simulink model "feedback_plant"  (R2024a)
settings: Solver=FixedStepAuto  StartTime=0.0  StopTime=Inf  FixedStep=5e-6  MaxStep=0.1  RelTol=1e-3  EnableMultiTasking=on
libraries: simulink x2
settings Model: ModifiedByFormat=The MathWorks Inc.  ExtModeTrigDuration=8  Creator=The MathWorks, Inc.  LastModifiedBy=The MathWorks Inc.
settings SolverCC: AlgebraicLoopSolver=TrustRegion
settings DataIOCC: SaveFormat=Array  ReturnWorkspaceOutputs=off
settings OptimizationCC: DefaultUnderspecifiedDataType=single  EnhancedBackFolding=on  PassReuseOutputArgsAs=Individual arguments  ExpressionDepthLimit=2147483647  MaxStackSize=1024  OptimizeBlockOrder=speed  DifferentSizesBufferReuse=on  OptimizationCustomize=off  EfficientTunableParamExpr=on
settings DebuggingCC: UnderspecifiedInitializationDetection=Classic  MergeDetectMultiDrivingBlocksExec=none  SolverPrmCheckMsg=warning  ParameterTunabilityLossMsg=error  FcnCallInpInsideContextMsg=warning  UnconnectedInputMsg=warning  UnconnectedOutputMsg=warning  UnconnectedLineMsg=warning  AllowSymbolicDim=off  StateNameClashWarn=warning  SFUnexpectedBacktrackingDiag=warning  SFNoUnconditionalDefaultTransitionDiag=warning  SFExecutionAtInitializationDiag=none  ArithmeticOperatorsInVariantConditions=warning
settings HardwareCC: ProdBitPerChar=16  ProdBitPerInt=16  ProdBitPerPointer=32  ProdBitPerSizeT=32  ProdBitPerPtrDiffT=32  ProdLargestAtomicInteger=Integer  ProdLargestAtomicFloat=None  ProdWordSize=16  ProdLongLongMode=on  ProdHWDeviceType=Texas Instruments->C2000  HardwareBoardFeatureSet=SoCBlockset
settings ModelReferenceCC: EnableRefExpFcnMdlSchedulingChecks=on  PropagateSignalLabelsOutOfModel=off
settings SFSimCC: SimUseLocalCustomCode=off  MATLABDynamicMemAlloc=off  CustomCodeUndefinedFunction=UseInterfaceOnly
settings RTWCC: Description=Embedded Coder  SystemTargetFile=ert.tlc  HardwareBoard=TI Delfino F28379D LaunchPad  TemplateMakefile=ert_default_tmf  RTWUseLocalCustomCode=off  Toolchain=Texas Instruments Code Composer Studio (C2000)  CodeProfilingSaveOptions=MetricsOnly  GPUComputeCapability=3.5
settings CodeAppCC: ForceParamTrailComments=on  IgnoreCustomStorageClasses=off  OperatorAnnotations=on  SimulinkDataObjDesc=on  SFDataObjDesc=on  InsertBlockDesc=on
settings ERTTargetCC: CodeReplacementLibrary=TI C28x  SupportContinuousTime=on  ExtModeTransport=4  ExtModeStaticAlloc=on  ExtModeAutomaticAllocSize=off  ExtModeStaticAllocSize=10000  ExtModeMexFile=ext_xcp  ExtModeIntrfLevel=Level2 - Open
settings ConfigComp: CovMetricSettings=dw  CovSaveCumulativeToWorkspaceVar=on  CovSaveSingleToWorkspaceVar=on  CovExternalEMLEnable=off  CovSFcnEnable=off

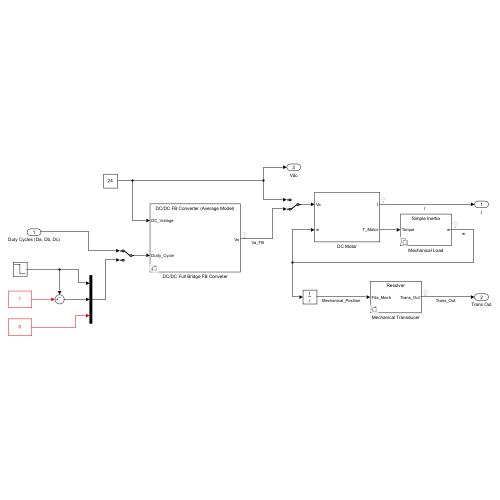
[thumbnail: Simulink's stored preview of the top-level diagram]
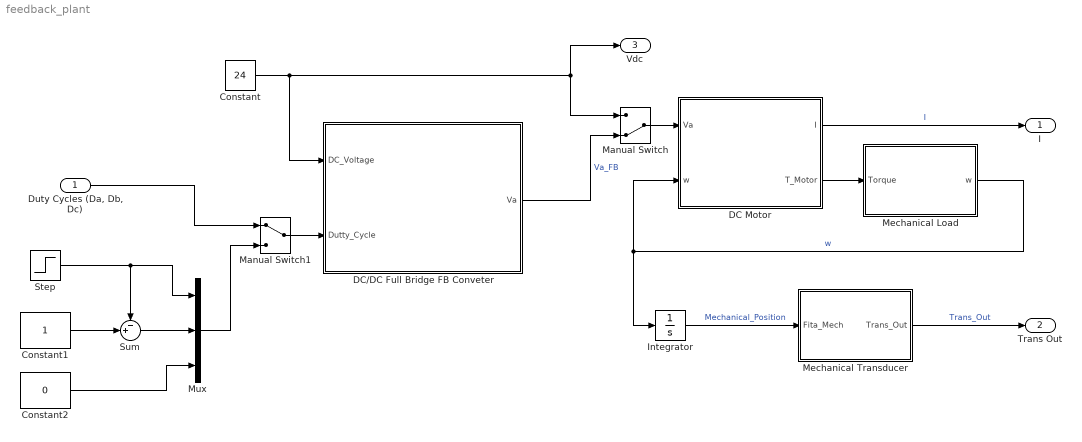
== system feedback_plant ==
  "Duty Cycles (Da, Db, Dc)" : Inport  PortDimensions=3
  Constant : Constant  Value=24
  Constant1 : Constant  OutDataTypeStr=Inherit: Inherit via back propagation  SampleTime=-1
  Constant2 : Constant  Value=0  OutDataTypeStr=Inherit: Inherit via back propagation  SampleTime=-1
  DC Motor : Subsystem  mask{R=705e-3, L=9.05e-3, Kf=3.8089}
      mask prompts: R "Resistance of the armature Ra [Ohms]:"; L "Inductance of the armature La [H]:"; Kf "Torque constant [Kf]:"
      mask DialogControl DescTextVar Prompt: This is the model of a Permanent Magnet DC Motor.
  DC/DC Full Bridge FB Conveter : Subsystem  Variant=on
  Integrator : Integrator
  Manual Switch : ManualSwitch  CurrentSetting=0
  Manual Switch1 : ManualSwitch
  Mechanical Load : Subsystem  Variant=on
  Mechanical Transducer : Subsystem  Variant=on
  Mux : Mux  Inputs=3
  Step : Step  Time=0.1  Before=0.6  After=0.4  SampleTime=0
  Sum : Sum  Inputs=-+|
  I : Outport
  Trans Out : Outport  Port=2
  Vdc : Outport  Port=3
  wires:
  DC Motor/1(I) -> I/1  "I"
  DC Motor/2(T_Motor) -> Mechanical Load/1(Torque)
  Mechanical Load/1(w) -> DC Motor/2(w), Integrator/1  "w"
  Manual Switch/1 -> DC Motor/1(Va)
  Constant/1 -> Vdc/1, Manual Switch/1, DC/DC Full Bridge FB Conveter/1(DC_Voltage)
  DC/DC Full Bridge FB Conveter/1(Va) -> Manual Switch/2  "Va_FB"
  Manual Switch1/1 -> DC/DC Full Bridge FB Conveter/2(Dutty_Cycle)
  "Duty Cycles (Da, Db, Dc)"/1 -> Manual Switch1/1
  Step/1 -> Mux/1, Sum/1
  Constant1/1 -> Sum/2
  Sum/1 -> Mux/2
  Mux/1 -> Manual Switch1/2
  Constant2/1 -> Mux/3
  Mechanical Transducer/1(Trans_Out) -> Trans Out/1  "Trans_Out"
  Integrator/1 -> Mechanical Transducer/1(Fita_Mech)  "Mechanical_Position"

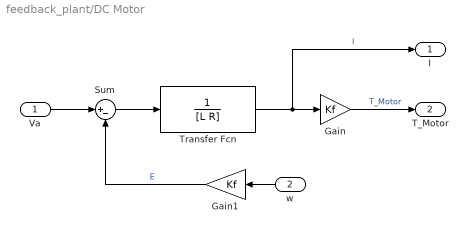
== system feedback_plant/DC Motor ==
  Va : Inport
  w : Inport  Port=2
  Gain : Gain  Gain=Kf
  Gain1 : Gain  Gain=Kf
  Sum : Sum  Inputs=|+-
  Transfer Fcn : TransferFcn  Denominator=[L R]
  I : Outport
  T_Motor : Outport  Port=2
  wires:
  Transfer Fcn/1 -> I/1, Gain/1  "I"
  Gain/1 -> T_Motor/1  "T_Motor"
  Sum/1 -> Transfer Fcn/1
  Gain1/1 -> Sum/2  "E"
  Va/1 -> Sum/1
  w/1 -> Gain1/1

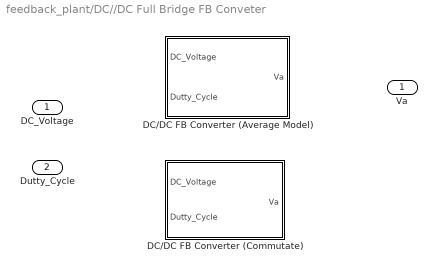
== system feedback_plant/DC//DC Full Bridge FB Conveter ==
  DC_Voltage : Inport
  Dutty_Cycle : Inport  Port=2
  DC/DC FB Converter (Average Model) : Subsystem  VariantControl=true
  DC/DC FB Converter (Commutate) : Subsystem  VariantControl=false
  Va : Outport

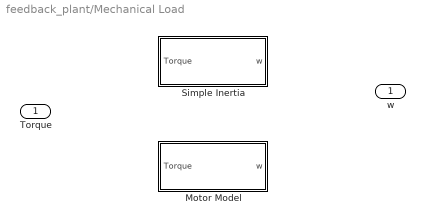
== system feedback_plant/Mechanical Load ==
  Torque : Inport
  Motor Model : Subsystem  VariantControl=false
  Simple Inertia : Subsystem  VariantControl=true  mask{f=0.0035, J=0.5}
      mask prompts: f "Friction coefficient:"; J "Inertia [Kg·m^2/s]:"
      mask DialogControl DescTextVar Prompt: This is the model of a simple Inertia with friction:
  w : Outport

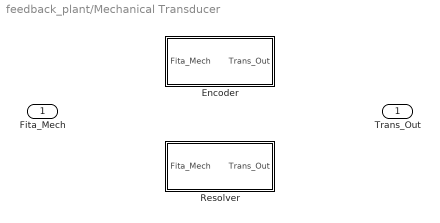
== system feedback_plant/Mechanical Transducer ==
  Fita_Mech : Inport
  Encoder : Subsystem  VariantControl=false
  Resolver : Subsystem  VariantControl=true
  Trans_Out : Outport

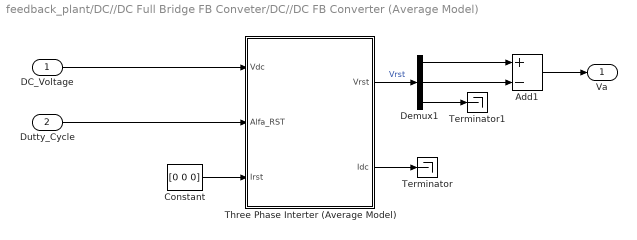
== system feedback_plant/DC//DC Full Bridge FB Conveter/DC//DC FB Converter (Average Model) ==
  DC_Voltage : Inport
  Dutty_Cycle : Inport  Port=2
  Add1 : Sum  Inputs=+-
  Constant : Constant  Value=[0 0 0]
  Demux1 : Demux  Outputs=3
  Terminator : Terminator
  Terminator1 : Terminator
  Three Phase Interter (Average Model) : Subsystem  VariantControl=VSS_TPH_INV_V0
  Va : Outport
  wires:
  Add1/1 -> Va/1
  DC_Voltage/1 -> Three Phase Interter (Average Model)/1(Vdc)
  Dutty_Cycle/1 -> Three Phase Interter (Average Model)/2(Alfa_RST)
  Constant/1 -> Three Phase Interter (Average Model)/3(Irst)
  Three Phase Interter (Average Model)/2(Idc) -> Terminator/1
  Three Phase Interter (Average Model)/1(Vrst) -> Demux1/1  "Vrst"
  Demux1/1 -> Add1/1
  Demux1/2 -> Add1/2
  Demux1/3 -> Terminator1/1

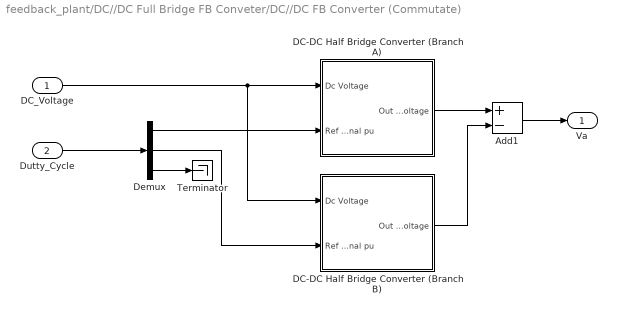
== system feedback_plant/DC//DC Full Bridge FB Conveter/DC//DC FB Converter (Commutate) ==
  DC_Voltage : Inport
  Dutty_Cycle : Inport  Port=2
  Add1 : Sum  Inputs=+-
  DC-DC Half Bridge Converter (Branch A) : Subsystem  mask{F=7}
      mask prompts: F "Commutation Frequency (kHz):"
  DC-DC Half Bridge Converter (Branch B) : Subsystem  mask{F=7}
      mask prompts: F "Commutation Frequency (kHz):"
  Demux : Demux  Outputs=3
  Terminator : Terminator
  Va : Outport
  wires:
  Add1/1 -> Va/1
  Demux/1 -> DC-DC Half Bridge Converter (Branch A)/2(Ref Signal pu)
  DC-DC Half Bridge Converter (Branch B)/1(Out Voltage) -> Add1/2
  Dutty_Cycle/1 -> Demux/1
  Demux/2 -> DC-DC Half Bridge Converter (Branch B)/2(Ref Signal pu)
  DC-DC Half Bridge Converter (Branch A)/1(Out Voltage) -> Add1/1
  DC_Voltage/1 -> DC-DC Half Bridge Converter (Branch A)/1(Dc Voltage), DC-DC Half Bridge Converter (Branch B)/1(Dc Voltage)
  Demux/3 -> Terminator/1

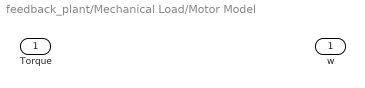
== system feedback_plant/Mechanical Load/Motor Model ==
  Torque : Inport
  w : Outport

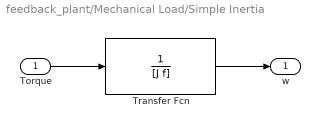
== system feedback_plant/Mechanical Load/Simple Inertia ==
  Torque : Inport
  Transfer Fcn : TransferFcn  Denominator=[J f]
  w : Outport
  wires:
  Torque/1 -> Transfer Fcn/1
  Transfer Fcn/1 -> w/1

== system feedback_plant/Mechanical Transducer/Encoder ==
  Fita_Mech : Inport
  Trans_Out : Outport
  wires:
  Fita_Mech/1 -> Trans_Out/1

== system feedback_plant/Mechanical Transducer/Resolver ==
  Fita_Mech : Inport
  Trans_Out : Outport
  wires:
  Fita_Mech/1 -> Trans_Out/1

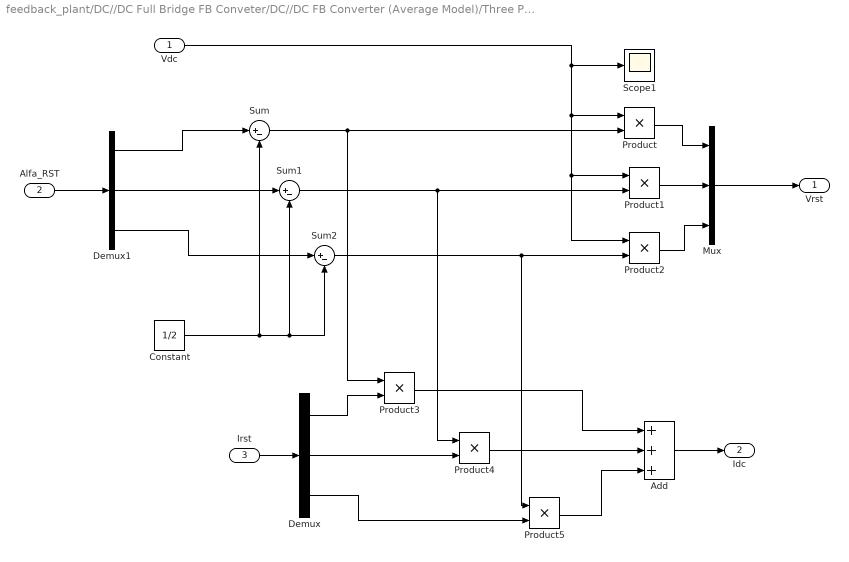
== system feedback_plant/DC//DC Full Bridge FB Conveter/DC//DC FB Converter (Average Model)/Three Phase Interter (Average Model) ==
  Vdc : Inport
  Alfa_RST : Inport  Port=2
  Irst : Inport  Port=3
  Add : Sum  Inputs=+++
  Constant : Constant  Value=1/2
  Demux : Demux  Outputs=3
  Demux1 : Demux  Outputs=3
  Mux : Mux  Inputs=3
  Product{,1..5} (6 alike) : Product
  Scope1 : Scope
  Sum : Sum  Inputs=|+-
  Sum1 : Sum  Inputs=|+-
  Sum2 : Sum  Inputs=|+-
  Vrst : Outport
  Idc : Outport  Port=2
  wires:
  Add/1 -> Idc/1
  Product5/1 -> Add/3
  Vdc/1 -> Scope1/1, Product1/1, Product2/1, Product/1
  Demux1/1 -> Sum/1
  Constant/1 -> Sum/2, Sum1/2, Sum2/2
  Product4/1 -> Add/2
  Sum1/1 -> Product4/1, Product1/2
  Product3/1 -> Add/1
  Sum/1 -> Product3/1, Product/2
  Product1/1 -> Mux/2
  Product2/1 -> Mux/3
  Sum2/1 -> Product5/1, Product2/2
  Product/1 -> Mux/1
  Demux1/2 -> Sum1/1
  Demux1/3 -> Sum2/1
  Demux/2 -> Product4/2
  Alfa_RST/1 -> Demux1/1
  Demux/3 -> Product5/2
  Demux/1 -> Product3/2
  Irst/1 -> Demux/1
  Mux/1 -> Vrst/1

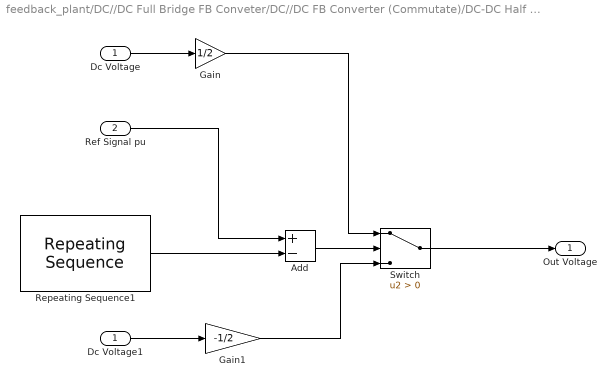
== system feedback_plant/DC//DC Full Bridge FB Conveter/DC//DC FB Converter (Commutate)/DC-DC Half Bridge Converter (Branch A) ==
  Dc Voltage : Inport
  Ref Signal pu : Inport  Port=2
  Add : Sum  Inputs=+-
  Dc Voltage1 : InportShadow
  Gain : Gain  Gain=1/2
  Gain1 : Gain  Gain=-1/2
  Repeating Sequence1 : simulink/Sources/Repeating Sequence  rep_seq_t=[0 a b]  rep_seq_y=[0 c d]  mask(Repeating table){F=F, Trig=Triangular}
      mask prompts: F "Enter the commutation Frequency (KHz):"; Trig "Select between Saw Tooth/Triangular:"
      mask init:
      | T =  1 / (F * 1000);
      | if (Trig == 1)
      |     % This mean the user has selected Saw Tooth Waveform
      |     a = T/2;
      |     b = T;
      |     c = 1/2;
      |     d = 1;
      | else
      |     % This mean the user has selected Triangular Waveform
      |     a = T/2;
      |     b = T;
      |     c = 1;
      |     d = 0;
      | end
      mask TypeOptions Trig: Saw Tooth | Triangular
  Switch : Switch  Criteria=u2 > Threshold  SaturateOnIntegerOverflow=off  InputSameDT=off
  Out Voltage : Outport
  wires:
  Add/1 -> Switch/2
  Repeating Sequence1/1 -> Add/2
  Dc Voltage1/1 -> Gain1/1
  Switch/1 -> Out Voltage/1
  Dc Voltage/1 -> Gain/1
  Gain/1 -> Switch/1
  Gain1/1 -> Switch/3
  Ref Signal pu/1 -> Add/1

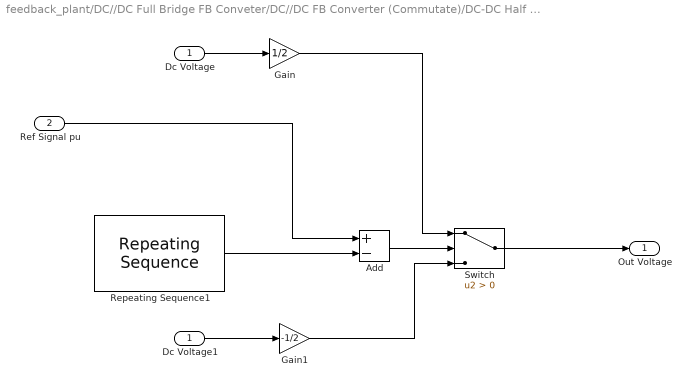
== system feedback_plant/DC//DC Full Bridge FB Conveter/DC//DC FB Converter (Commutate)/DC-DC Half Bridge Converter (Branch B) ==
  Dc Voltage : Inport
  Ref Signal pu : Inport  Port=2
  Add : Sum  Inputs=+-
  Dc Voltage1 : InportShadow
  Gain : Gain  Gain=1/2
  Gain1 : Gain  Gain=-1/2
  Repeating Sequence1 : simulink/Sources/Repeating Sequence  rep_seq_t=[0 a b]  rep_seq_y=[0 c d]  mask(Repeating table){F=F, Trig=Triangular}
      mask prompts: F "Enter the commutation Frequency (KHz):"; Trig "Select between Saw Tooth/Triangular:"
      mask init: same as feedback_plant/DC//DC Full Bridge FB Conveter/DC//DC FB Converter (Commutate)/DC-DC Half Bridge Converter (Branch A)/Repeating Sequence1
      mask TypeOptions Trig: Saw Tooth | Triangular
  Switch : Switch  Criteria=u2 > Threshold  SaturateOnIntegerOverflow=off  InputSameDT=off
  Out Voltage : Outport
  wires:
  Ref Signal pu/1 -> Add/1
  Gain1/1 -> Switch/3
  Gain/1 -> Switch/1
  Dc Voltage/1 -> Gain/1
  Switch/1 -> Out Voltage/1
  Dc Voltage1/1 -> Gain1/1
  Repeating Sequence1/1 -> Add/2
  Add/1 -> Switch/2
